simulink model "Cascaded_Water_Tanks_Simulink_2022a"  (R2022a)
settings: Solver=VariableStepAuto  StartTime=0.0  StopTime=600  FixedStep=1  RelTol=1e-3
values from neighbouring files (symbols this model uses):
  a0 = R_pipe2    (= 1701.41579261)    [Cascaded_Water_Tanks_final.m]
  b0 = 1    [Cascaded_Water_Tanks_final.m]
  b1 = A_tank1*R_pipe1 + A_tank2*R_pipe2    (= 1503.32494353)    [Cascaded_Water_Tanks_final.m]
  b2 = A_tank1*A_tank2*R_pipe1*R_pipe2    (= 564996.47146)    [Cascaded_Water_Tanks_final.m]
  q_in = 3.4e-3    (= 0.0034)    [Cascaded_Water_Tanks_final.m]
libraries: slpidlib x1
settings Model: Creator=const  LastModifiedBy=const
settings ModelReferenceCC: EnableRefExpFcnMdlSchedulingChecks=off
settings RTWCC: Description=Generic Real-Time Target

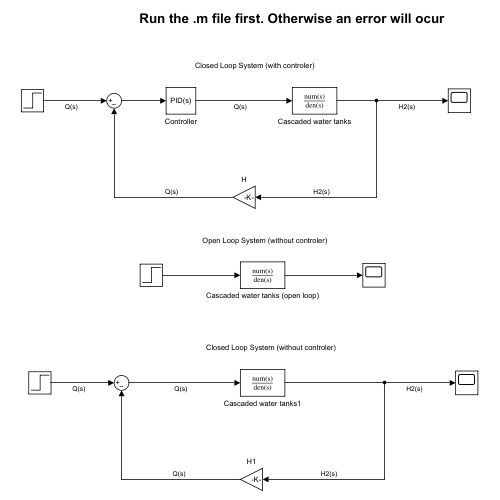
[thumbnail: Simulink's stored preview of the top-level diagram]
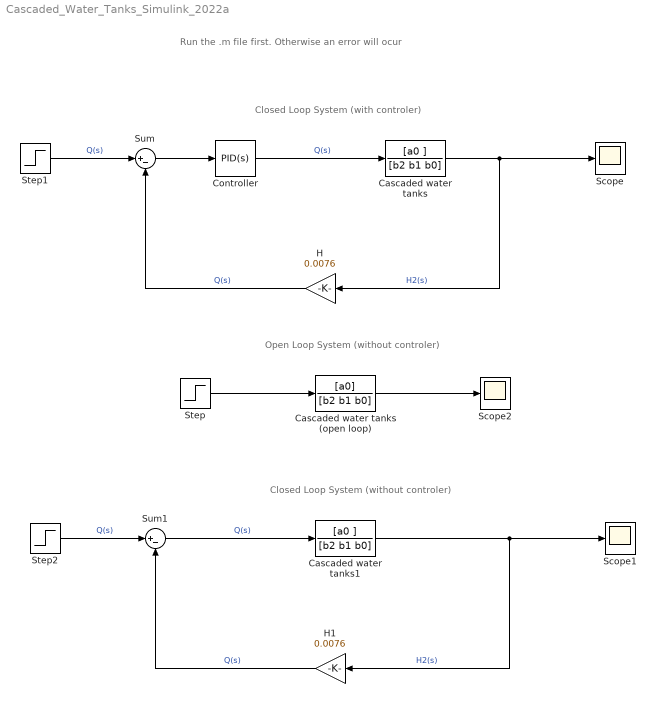
== system Cascaded_Water_Tanks_Simulink_2022a ==
  note: Closed Loop System (without controler)
  note: Run the .m file first. Otherwise an error will ocur
  note: Closed Loop System (with controler)
  note: Open Loop System (without controler)
  Cascaded water tanks : TransferFcn  Numerator=[a0 ]  Denominator=[b2 b1 b0]
  Cascaded water tanks (open loop) : TransferFcn  Numerator=[a0]  Denominator=[b2 b1 b0]
  Cascaded water tanks1 : TransferFcn  Numerator=[a0 ]  Denominator=[b2 b1 b0]
  Controller : slpidlib/PID Controller  Controller=PID  Form=Parallel  TimeDomain=Continuous-time  UseExternalTs=off  SampleTime=-1  IntegratorMethod=Forward Euler  FilterMethod=Forward Euler  ControllerParametersSource=internal  P=3.92/2.6  I=1.23e-3  UseKiTs=off  D=6.265e2  N=100  UseFilter=on  TunerSelectOption=Transfer Function Based (PID Tuner App)  InitialConditionSource=internal  InitialConditionForIntegrator=0  InitialConditionForFilter=0  DifferentiatorICPrevScaledInput=0  ExternalReset=none  TrackingMode=off  Kt=1  LimitOutput=off  SatLimitsSource=internal  UpperSaturationLimit=inf  LowerSaturationLimit=-inf  LinearizeAsGain=on  AntiWindupMode=none  Kb=1  POutMin=[]  POutMax=[]  IOutMin=[]  IOutMax=[]  DOutMin=[]  DOutMax=[]  NOutMin=[]  NOutMax=[]  SumOutMin=[]  SumOutMax=[]  SaturationOutMin=[]  SaturationOutMax=[]  PParamMin=[]  PParamMax=[]  IParamMin=[]  IParamMax=[]  DParamMin=[]  DParamMax=[]  NParamMin=[]  NParamMax=[]  KbParamMin=[]  KbParamMax=[]  KtParamMin=[]  KtParamMax=[]  KbOutMin=[]  KbOutMax=[]  KtOutMin=[]  KtOutMax=[]  IntegratorOutMin=[]  IntegratorOutMax=[]  FilterOutMin=[]  FilterOutMax=[]  SumI1OutMin=[]  SumI1OutMax=[]  SumI2OutMin=[]  SumI2OutMax=[]  SumI3OutMin=[]  SumI3OutMax=[]  SumI4OutMin=[]  SumI4OutMax=[]  SumDOutMin=[]  SumDOutMax=[]  DifferentiatorOutMin=[]  DifferentiatorOutMax=[]  FilterDiffOutCoefMin=[]  FilterDiffOutCoefMax=[]  ReciprocalOutMin=[]  ReciprocalOutMax=[]  SumDenOutMin=[]  SumDenOutMax=[]  SumNumOutMin=[]  SumNumOutMax=[]  DivideOutMin=[]  DivideOutMax=[]  UdiffTsProdOutMin=[]  UdiffTsProdOutMax=[]  NTsProdOutMin=[]  NTsProdOutMax=[]  UintegralTsProdOutMin=[]  UintegralTsProdOutMax=[]  UngainTsProdOutMin=[]  UngainTsProdOutMax=[]  IntegratorContinuousStateAttributes=''  IntegratorStateMustResolveToSignalObject=off  IntegratorRTWStateStorageClass=Auto  FilterContinuousStateAttributes=''  FilterStateMustResolveToSignalObject=off  FilterRTWStateStorageClass=Auto  ParallelPVariant=InternalParameters  IdealPVariant=Disabled  IVariant=InternalParameters  DVariant=InternalParameters  IntegratorVariant=Continuous  SatVariant=Disabled  AWVariant=Passthrough  PCopyVariant=Disabled  TRVariant=Disabled  FdbkBlocksVariant=Forward  IdealPFdbkVariant=Disabled  SatFdbkVariant=Disabled  DerivativeFilterVariant=ContFilter  NVariant=InternalParameters  NCopyVariant=Disabled  FilterICVariant=InternalICsFilter  IntegratorICVariant=InternalICs  ExternalResetVariant=Disabled  TRSumVariant=Passthrough  SumFdbkVariant=Disabled  SumVariant=Sum_PID  TsampFilterVariant=InternalTs  TsampNgainVariant=Passthrough  TsampIntegralVariant=Disabled_SignalSpec  ExternalSaturationOutDataTypeStr=Inherit: Same as second input
  H : Gain  Gain=0.0076
  H1 : Gain  Gain=0.0076
  Scope : Scope
  Scope1 : Scope
  Scope2 : Scope
  Step : Step  Time=0  After=q_in  SampleTime=0
  Step1 : Step  Time=0  After=q_in  SampleTime=0
  Step2 : Step  Time=0  After=q_in  SampleTime=0
  Sum : Sum  Inputs=|+-
  Sum1 : Sum  Inputs=|+-
  wires:
  Cascaded water tanks/1 -> H/1, Scope/1  "H2(s)"
  Step/1 -> Cascaded water tanks (open loop)/1
  Cascaded water tanks (open loop)/1 -> Scope2/1
  Controller/1 -> Cascaded water tanks/1  "Q(s)"
  Sum/1 -> Controller/1
  H/1 -> Sum/2  "Q(s)"
  Step1/1 -> Sum/1  "Q(s)"
  Step2/1 -> Sum1/1  "Q(s)"
  H1/1 -> Sum1/2  "Q(s)"
  Sum1/1 -> Cascaded water tanks1/1  "Q(s)"
  Cascaded water tanks1/1 -> Scope1/1, H1/1  "H2(s)"
